simulink model "DC_MOTOR_CONTROL_SIMULACION"  (R2022b)
settings: Solver=ode45  StartTime=0.0  StopTime=100  RelTol=1e-3
libraries: fod x3, SignalEditorBlockLib x1
settings Model: Creator=mario  LastModifiedBy=mario
settings SolverCC: ZeroCrossAlgorithm=Adaptive
settings DebuggingCC: IgnoredZcDiagnostic=none

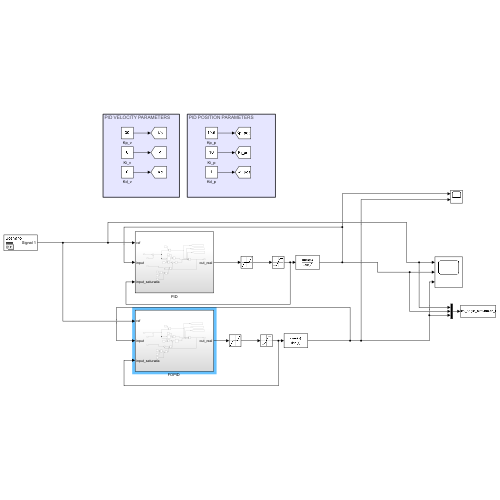
[thumbnail: Simulink's stored preview of the top-level diagram]
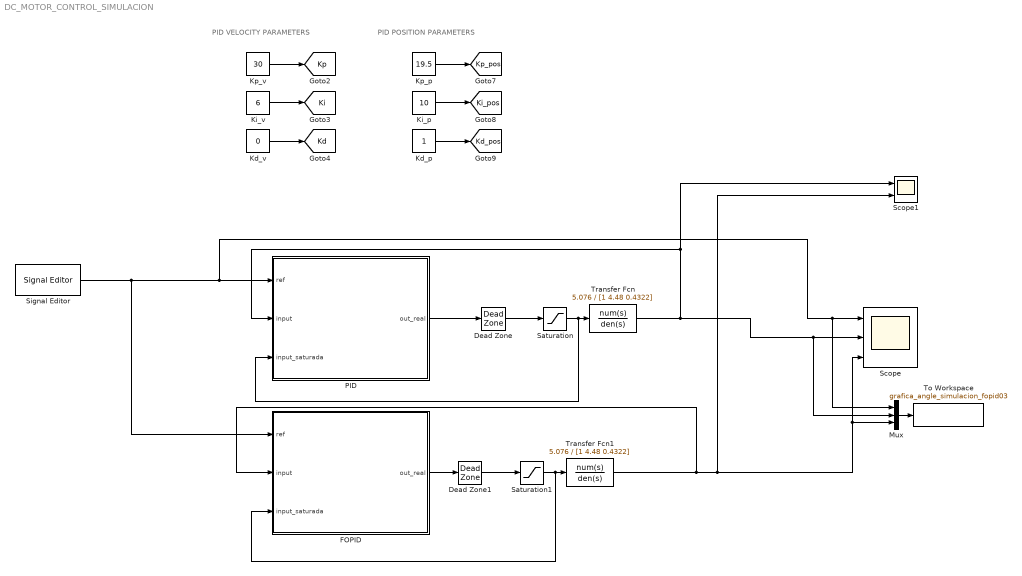
== system DC_MOTOR_CONTROL_SIMULACION ==
  note: PID VELOCITY PARAMETERS
  note: PID POSITION PARAMETERS
  Dead Zone : DeadZone  LowerValue=-70  UpperValue=70
  Dead Zone1 : DeadZone  LowerValue=-70  UpperValue=70
  "FOPID " : Subsystem
  Kd_p : Constant
  Kd_v : Constant  Value=0
  Ki_p : Constant  Value=10
  Ki_v : Constant  Value=6
  Kp_p : Constant  Value=19.5
  Kp_v : Constant  Value=30
  Mux : Mux  Inputs=3
  PID : Subsystem
  Saturation : Saturate  UpperLimit=255  LowerLimit=-255
  Saturation1 : Saturate  UpperLimit=255  LowerLimit=-255
  Scope : Scope  NumInputPorts=3
  Scope1 : Scope  NumInputPorts=2
  Signal Editor : SignalEditorBlockLib/Signal Editor  FileName=ANGLE_REFERENCE.mat  ActiveScenario=Scenario  ActiveSignal=Signal 1  IsBus=off  OutputBusObjectStr=Bus: BusObject  SampleTime=0  Interpolate=off  ZeroCross=off  OutputAfterFinalValue=Setting to zero  Unit=inherit  PreserveSignalName=on
  To Workspace : ToWorkspace  VariableName=grafica_angle_simulacion_fopid03  SampleTime=0.01
  Transfer Fcn : TransferFcn  Numerator=5.076  Denominator=[1 4.48 0.4322]
  Transfer Fcn1 : TransferFcn  Numerator=5.076  Denominator=[1 4.48 0.4322]
  tag scope: Kd=global, Kd_pos=global, Ki=global, Ki_pos=global, Kp=global, Kp_pos=global
  wires:
  Signal Editor/1 -> "FOPID "/1(ref), PID/1(ref), Mux/1, Scope/1
  PID/1(out_real) -> Dead Zone/1
  Dead Zone/1 -> Saturation/1
  Saturation/1 -> PID/3(input_saturada), Transfer Fcn/1
  Transfer Fcn/1 -> PID/2(input), Scope1/1, Mux/2, Scope/2
  "FOPID "/1(out_real) -> Dead Zone1/1
  Saturation1/1 -> Transfer Fcn1/1, "FOPID "/3(input_saturada)
  Transfer Fcn1/1 -> "FOPID "/2(input), Scope1/2, Mux/3, Scope/3
  Kp_v/1 -> [Kp]
  Ki_v/1 -> [Ki]
  Kp_p/1 -> [Kp_pos]
  Kd_v/1 -> [Kd]
  Kd_p/1 -> [Kd_pos]
  Ki_p/1 -> [Ki_pos]
  Dead Zone1/1 -> Saturation1/1
  Mux/1 -> To Workspace/1

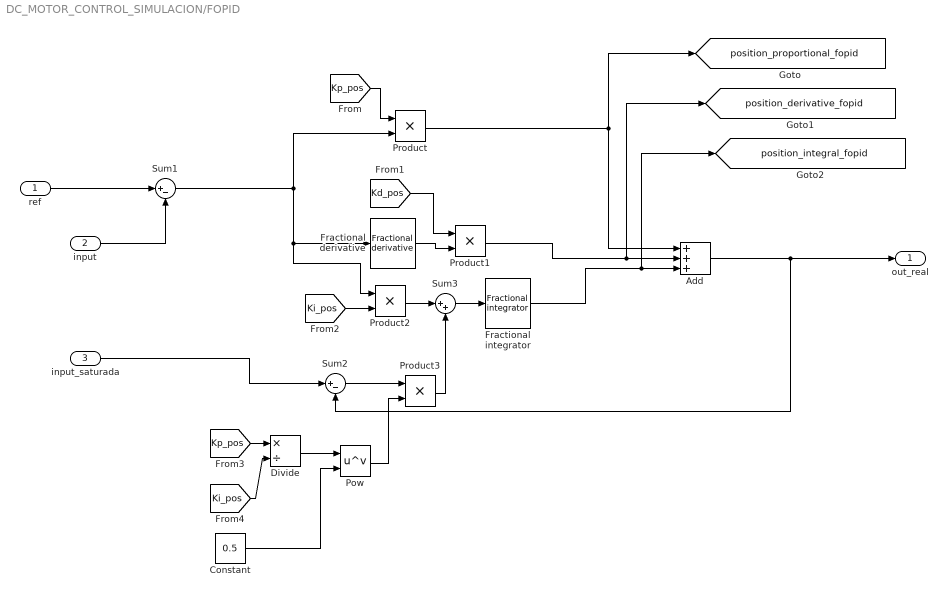
== system DC_MOTOR_CONTROL_SIMULACION/FOPID  ==
  ref : Inport
  input : Inport  Port=2
  input_saturada : Inport  Port=3
  Add : Sum  Inputs=+++
  Constant : Constant  Value=0.5
  Divide : Product  Inputs=*/
  Fractional derivative : fod/Fractional derivative  gam=0.95  ww=[0.1; 50]  n=5  nFod=off
      settings: SourceProductName=FOMCON Toolbox
  Fractional integrator : fod/Fractional integrator  gam=0.15  ww=[0.1; 50]  n=5  nFod=off
      settings: SourceProductName=FOMCON Toolbox
  Pow : Math  Operator=pow  SignedPower=on  RndMeth=Zero
  Product{,1..3} (4 alike) : Product
  Sum1 : Sum  Inputs=|+-
  Sum2 : Sum  Inputs=|+-
  Sum3 : Sum  Inputs=|++
  out_real : Outport
  tag scope: position_derivative_fopid=global, position_integral_fopid=global, position_proportional_fopid=global
  wires:
  ref/1 -> Sum1/1
  input/1 -> Sum1/2
  Add/1 -> Sum2/2, out_real/1
  Sum1/1 -> Product2/1, Fractional derivative/1, Product/2
  Product2/1 -> Sum3/1
  Sum3/1 -> Fractional integrator/1
  Sum2/1 -> Product3/1
  input_saturada/1 -> Sum2/1
  Fractional derivative/1 -> Product1/2
  [Kp_pos] -> Product/1
  [Kd_pos] -> Product1/1
  [Ki_pos] -> Product2/2
  [Kp_pos] -> Divide/1
  [Ki_pos] -> Divide/2
  Divide/1 -> Pow/1
  Constant/1 -> Pow/2
  Pow/1 -> Product3/2
  Product3/1 -> Sum3/2
  Fractional integrator/1 -> [position_integral_fopid], Add/3
  Product/1 -> Add/1, [position_proportional_fopid]
  Product1/1 -> [position_derivative_fopid], Add/2

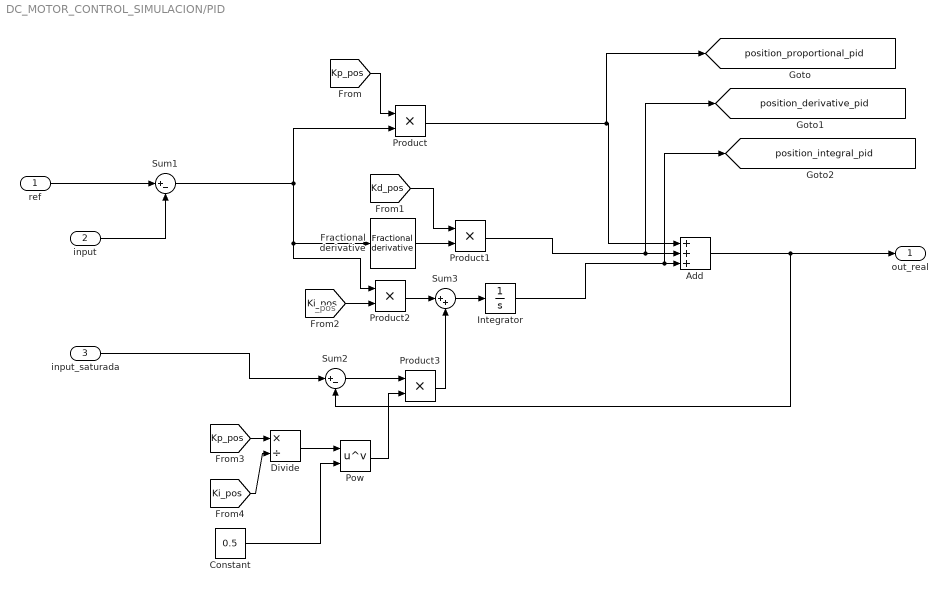
== system DC_MOTOR_CONTROL_SIMULACION/PID ==
  note: _pos
  ref : Inport
  input : Inport  Port=2
  input_saturada : Inport  Port=3
  Add : Sum  Inputs=+++
  Constant : Constant  Value=0.5
  Divide : Product  Inputs=*/
  Fractional derivative : fod/Fractional derivative  gam=1  ww=[0.1; 50]  n=5  nFod=off
      settings: SourceProductName=FOMCON Toolbox
  Integrator : Integrator
  Pow : Math  Operator=pow  SignedPower=on  RndMeth=Zero
  Product{,1..3} (4 alike) : Product
  Sum1 : Sum  Inputs=|+-
  Sum2 : Sum  Inputs=|+-
  Sum3 : Sum  Inputs=|++
  out_real : Outport
  tag scope: position_derivative_pid=global, position_integral_pid=global, position_proportional_pid=global
  wires:
  ref/1 -> Sum1/1
  input/1 -> Sum1/2
  Add/1 -> Sum2/2, out_real/1
  Product/1 -> [position_proportional_pid], Add/1
  Sum1/1 -> Fractional derivative/1, Product2/1, Product/2
  Product1/1 -> Add/2, [position_derivative_pid]
  Product2/1 -> Sum3/1
  Sum3/1 -> Integrator/1
  Sum2/1 -> Product3/1
  Integrator/1 -> [position_integral_pid], Add/3
  input_saturada/1 -> Sum2/1
  Fractional derivative/1 -> Product1/2
  [Kp_pos] -> Product/1
  [Kd_pos] -> Product1/1
  [Ki_pos] -> Product2/2
  [Kp_pos] -> Divide/1
  [Ki_pos] -> Divide/2
  Divide/1 -> Pow/1
  Constant/1 -> Pow/2
  Pow/1 -> Product3/2
  Product3/1 -> Sum3/2
